simulink model "examp1"  (Simulink 4.00)
settings: Solver=ode45  StartTime=0.0  StopTime=10.0  RelTol=1e-3
settings Model: LastModifiedBy=bobov

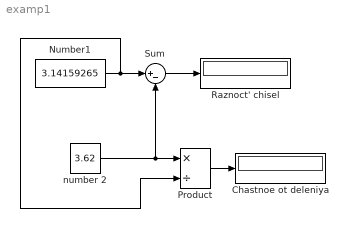
== system examp1 ==
  Chastnoe ot deleniya : Display
      settings: Format=short
  Number1 : Constant  Value=3.14159265
  Product : Product  Inputs=*/  Multiplication=Element-wise(.*)  SaturateOnIntegerOverflow=on
  Raznoct' chisel : Display
      settings: Format=short
  Sum : Sum  Inputs=|+-  SaturateOnIntegerOverflow=on
  number 2 : Constant  Value=3.62
  wires:
  Number1/1 -> Sum/1, Product/2
  Sum/1 -> Raznoct' chisel/1
  number 2/1 -> Sum/2, Product/1
  Product/1 -> Chastnoe ot deleniya/1
